simulink model "DC_mOTOR_VERSION2"  (R2022a)
settings: Solver=VariableStepAuto  StartTime=0.0  StopTime=10.0  RelTol=1e-3
undefined symbols (not defined in the file): sigbuilder_block
settings Model: Creator=DELL  LastModifiedBy=DELL

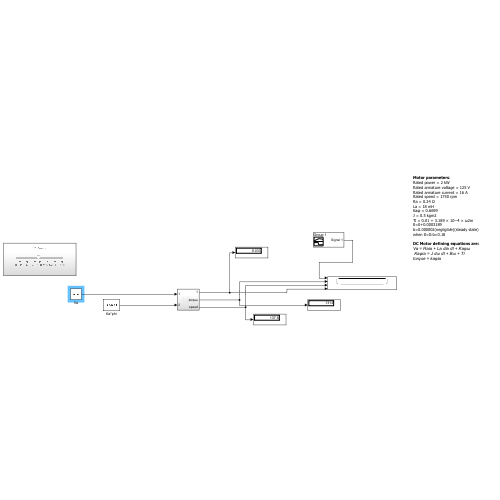
[thumbnail: Simulink's stored preview of the top-level diagram]
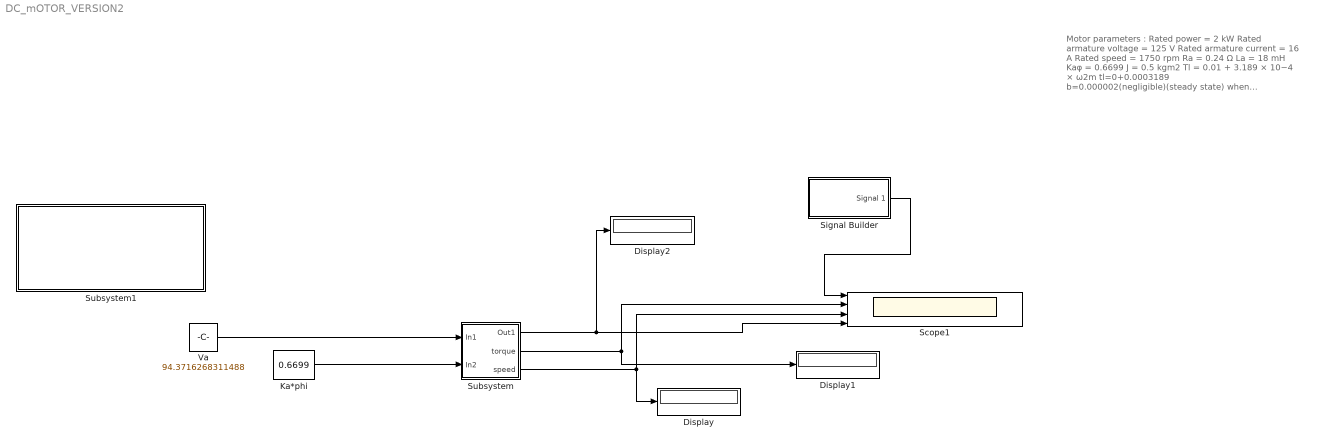
== system DC_mOTOR_VERSION2 ==
  note: Motor parameters :
      | Rated power = 2 kW
      | Rated armature voltage = 125 V
      | Rated armature current = 16 A
      | Rated speed = 1750 rpm
      | Ra = 0.24 Ω
      | La = 18 mH
      | Kaφ = 0.6699
      | J = 0.5 kgm2
      | Tl = 0.01 + 3.189 × 10−4 × ω2m
      | tl=0+0.0003189
      | b=0.000002(negligible)(steady state)
      | when tl=0:b=0.18
      |
      | DC Motor defining equations are:
      | Va = Raia + La dia dt + Kaφω
      | Kaφia = J dω dt + Bω + Tl
      | torque = kaφia
  Display : Display
  Display1 : Display
  Display2 : Display
  Ka*phi : Constant  Value=0.6699
  Scope1 : Scope  NumInputPorts=4
  Signal Builder : Subsystem  Tag=STV Subsys  LoadFcn=sigbuilder_block('load');  StartFcn=sigbuilder_block('start');  StopFcn=sigbuilder_block('stop');  ClipboardFcn=sigbuilder_block('clipboard');  mask(Sigbuilder block){tuvar=[0:10]}
      mask help: Simulink:masks:SigbuilderBlock_MD
      mask init:
      | if ~strcmp(get_param(bdroot(gcbh),'SimulationStatus'),'stopped') tuvar = sigbuilder_block('maskInit'); end
      settings: CopyFcn=sigbuilder_block('copy');  DeleteFcn=sigbuilder_block('delete');  ModelCloseFcn=sigbuilder_block('modelClose');  PreSaveFcn=sigbuilder_block('preSave');  PauseFcn=sigbuilder_block('pause');  ContinueFcn=sigbuilder_block('continue');  NameChangeFcn=sigbuilder_block('namechange');  OpenFcn=sigbuilder_block('open',[437.6 153 550.4 359.25 ]);  CloseFcn=sigbuilder_block('close');
      mask Display: plot(0, 0, 100, 100,[2, 2, 32, 32, 2], [68, 8, 8, 68, 68],[32, 2], [38, 38], [32, 19, 2],[53, 60, 44], [32, 17, 17, 2],[16, 16, 31, 31]);txt = getActiveGroup(gcbh);text(2, 100, txt,'verticalAlignment', 'top');
  Subsystem : Subsystem
  Subsystem1 : Subsystem
  Va : Constant  Value=94.3716268311488
  wires:
  Subsystem/3(speed) -> Display/1, Scope1/3
  Va/1 -> Subsystem/1(In1)
  Subsystem/1(Out1) -> Display2/1, Scope1/4
  Subsystem/2(torque) -> Display1/1, Scope1/2
  Ka*phi/1 -> Subsystem/2(In2)
  Signal Builder/1(Signal 1) -> Scope1/1

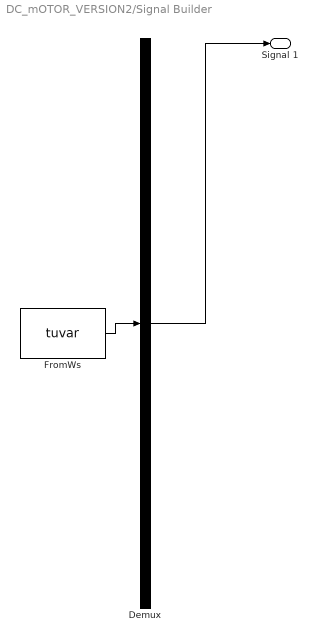
== system DC_mOTOR_VERSION2/Signal Builder ==
  Demux : Demux  Tag=STV Demux  Outputs=1
      settings: DisplayOption=none
  FromWs : FromWorkspace  Tag=STV FromWs  VariableName=tuvar
      SigBuilderData=|
      | common.afterFinalStr = 'Extrapolate'
      | common.sampleTime = 0
      | dataSet.timeRange = [0 10]
      | dataSet.name = 'Group 1'
      | sbobj.Groups.Name = 'Group 1'
      | sbobj.Groups.Signals.Name = 'Signal 1'
      | sbobj.Groups.Signals.XData = [0 4 4 6 6 10]
      | sbobj.Groups.Signals.YData = [0 0 1 1 0 0]
  Signal 1 : Outport  Tag=STV Outport
  wires:
  Demux/1 -> Signal 1/1
  FromWs/1 -> Demux/1

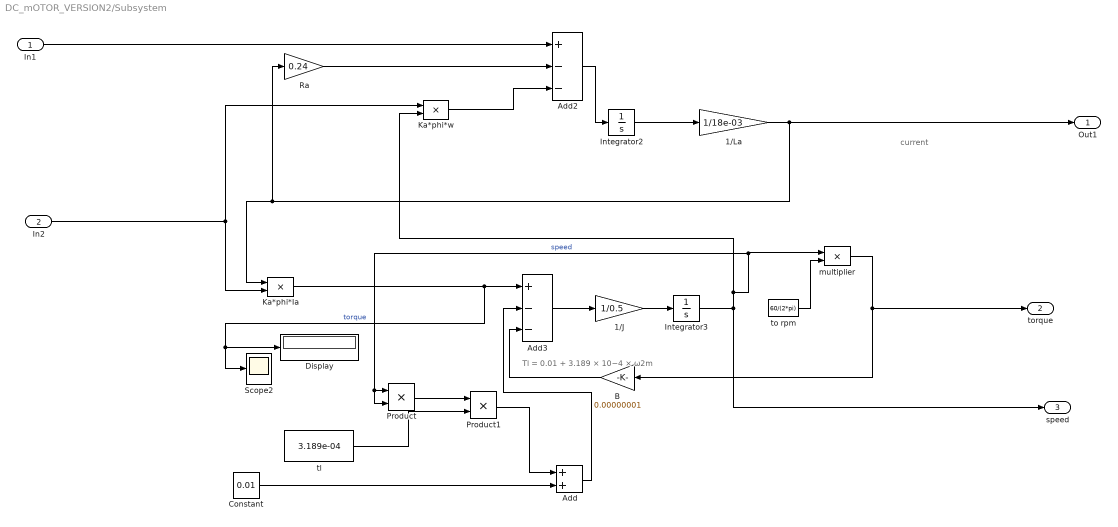
== system DC_mOTOR_VERSION2/Subsystem ==
  note: current
  note: Tl = 0.01 + 3.189 × 10−4 × ω2m
  In1 : Inport
  In2 : Inport  Port=2
  1/J : Gain  Gain=1/0.5
  1/La : Gain  Gain=1/18e-03
  Add : Sum
  Add2 : Sum  Inputs=+--
  Add3 : Sum  Inputs=+--
  B : Gain  Gain=0.00000001
  Constant : Constant  Value=0.01
  Display : Display
  Integrator2 : Integrator
  Integrator3 : Integrator
  Ka*phi*Ia : Product
  Ka*phi*w : Product
  Product : Product
  Product1 : Product
  Ra : Gain  Gain=0.24
  Scope2 : Scope
  multiplier : Product
  tl : Constant  Value=3.189e-04
  to rpm : Constant  Value=60/(2*pi)
  Out1 : Outport
  torque : Outport  Port=2
  speed : Outport  Port=3
  wires:
  Add2/1 -> Integrator2/1
  B/1 -> Add3/3
  Integrator3/1 -> speed/1, Ka*phi*w/2, Product/2, Product/1, multiplier/1  "speed"
  Ka*phi*w/1 -> Add2/3
  Add3/1 -> 1/J/1
  1/J/1 -> Integrator3/1
  tl/1 -> Product1/2
  Ra/1 -> Add2/2
  Ka*phi*Ia/1 -> Display/1, Scope2/1, Add3/1  "torque"
  Product1/1 -> Add/1
  In2/1 -> Ka*phi*Ia/2, Ka*phi*w/1
  multiplier/1 -> torque/1, B/1
  In1/1 -> Add2/1
  to rpm/1 -> multiplier/2
  1/La/1 -> Ka*phi*Ia/1, Ra/1, Out1/1
  Constant/1 -> Add/2
  Integrator2/1 -> 1/La/1
  Add/1 -> Add3/2
  Product/1 -> Product1/1

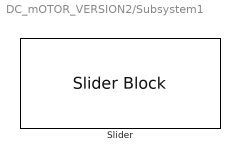
== system DC_mOTOR_VERSION2/Subsystem1 ==
  Slider : SliderBlock  ScaleMax=200
